simulink model "MultirotorSimPx4v1_8ContMatrix"  (R2018b)
settings: Solver=ode45  StartTime=0.0  StopTime=Simulation.T_END  MaxStep=Simulation.TS_MAX  RelTol=1e-3  EnableMultiTasking=on
PreLoadFcn:
  | % InitializeParameters;
undefined symbols (not defined in the file): Ctrl, Initial, Kpid, Uav, Wind
libraries: QuaternionLibrary x13, simulink x5, simulink_extras x4
(part 1 of 2)
settings Model: Creator=jban039  LastModifiedBy=jban039
settings DataIOCC: Decimation=10  ExternalInput=getinputstruct(op1(2))  InitialState=getstatestruct(op)  SaveFormat=StructureWithTime  ReturnWorkspaceOutputs=on  OutputTimes=Simulation.T_OUT
settings OptimizationCC: LifeSpan=inf
settings DebuggingCC: ReadBeforeWriteMsg=DisableAll  WriteAfterWriteMsg=DisableAll  WriteAfterReadMsg=DisableAll  MultiTaskDSMMsg=none  UnconnectedLineMsg=none  AllowSymbolicDim=off  SFUnexpectedBacktrackingDiag=warning  SFNoUnconditionalDefaultTransitionDiag=warning  SFExecutionAtInitializationDiag=none
settings ModelReferenceCC: UpdateModelReferenceTargets=IfOutOfDate  ModelReferenceMinAlgLoopOccurrences=on  PropagateSignalLabelsOutOfModel=off
settings SFSimCC: SFSimEcho=off  SimUseLocalCustomCode=off
settings RTWCC: RTWUseLocalCustomCode=off
settings CodeAppCC: StateflowObjectComments=on
settings GRTTargetCC: TargetLangStandard=C89/C90 (ANSI)
settings ConfigComp: CovMetricSettings=dw  CovHtmlReporting=on  CovSaveCumulativeToWorkspaceVar=on  CovSaveSingleToWorkspaceVar=on  CovExternalEMLEnable=off

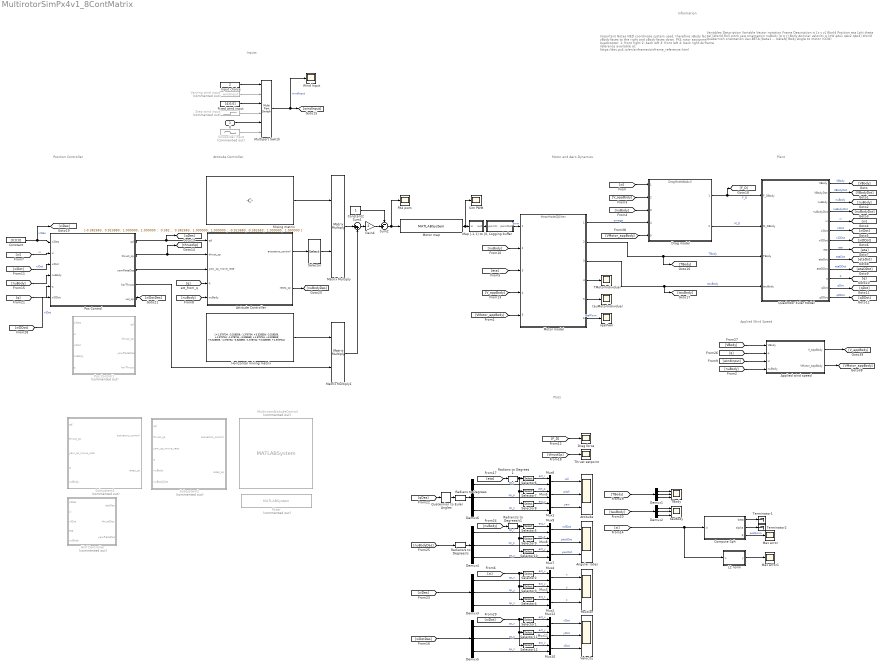
== system MultirotorSimPx4v1_8ContMatrix ==
  note: Plots
  note: Inputs
  note: Motor and Aero Dynamics
  note: Plant
  note: Attitude Controller
  note: Position Controller
  note: Applied Wind Speed
  note: Important Notes
      |
      | NED coordinate system used, therefore xBody faces forward, yBody faces to the right and zBody faces down.
      | PX4 rotor assignment for quadcopter:
      | 1: front right
      | 2: back left
      | 3: front left
      | 4: back right
      | Airframe reference available at:
      | https://dev.px4.io/en/airframes/airframe_reference.html
  note: Variables Description
      |
      | Variable
      | Vector notation
      | Frame
      | Description
      |
      | xi
      | [x y z]
      | World
      | Position
      |
      | eta
      | [phi theta psi]
      | World
      | Roll pitch yaw orientation
      |
      | nuBody
      | [p q r]
      | Body
      | Angular velocity
      |
      | q
      | [qW qAx1 qAx2 qAx3]
      | World
      | Quaternion orientation
      |
      | Uav.BETA
      | [beta1 ... betaN]
      | Body
      | Angle to motor (CCW)
  note: Information
  U : Inport  PortDimensions=3
  Angular rates : Scope  NumInputPorts=3
  Applied wind speed : Subsystem
  Attitude : Scope  NumInputPorts=3
  Attitude Controller : Subsystem
      mask Display: fprintf('MC_ATT_CONTROL\n\nCONTINUOUS')
  Compute Sph : MATLAB Function  TreatAsAtomicUnit=on
  Constant : Constant  Value=[0;0;0]
  Constant2 : Constant
  Demux{1..6} (6 alike) : Demux  Outputs=3
  Drag force : Scope
  Drag model : ModelReference  ModelNameDialog=DragModelAIAAv3  SimulationMode=Normal  ModelReferenceVersion=1.368
  Fixed wind input : Constant  Value=[4;0;0]
  Gain4 : Gain  Gain=2
  Hinf Controller : Subsystem  Commented=on
  Horizontal mixing matrix : Constant  Value=|
      | [+1.378734, -3.328559;
      |  -1.378734, +3.328559;
      |  -3.328559, +1.378734;
      |  -1.378734, -3.328559;
      |  +1.378734, +3.328559;
      |  +3.328559, -1.378734;
      |  -3.328559, -1.378734;
      |  +3.328559, +1.378734]
  Input choice : Constant  Value=2
  L2 norm : MATLAB Function  TreatAsAtomicUnit=on
  Logging buffer : Subsystem
  Map [-1,1] to [0,1] : Subsystem
  Matrix Multiply : Product  Multiplication=Matrix(*)
  Matrix Multiply1 : Product  Multiplication=Matrix(*)
  Max error : Scope
  Max error1 : Scope
  Mixer : MATLABSystem  Commented=on  SCDEnableBlockLinearizationSpecification=on  System=MultirotorMixer  airframeConfig=5  useHorThrust=0  outputSatStatus=0  SimulateUsing=Interpreted execution
      mask Type: MultirotorMixer
      mask Display:
      | disp(['MULTIROTOR' char(10) 'MIXER' char(10) 'octa_x']);
      | port_label('input',1,'actuatorsControl');
      | port_label('output',1,'px4PWM');
  Mixing matrix : Constant  Value=|
      | [-0.382683,  0.923880,  1.000000,  1.000000 ;
      |   0.382683, -0.923880,  1.000000,  1.000000 ;
      |  -0.923880,  0.382683, -1.000000,  1.000000 ;
      |  -0.382683, -0.923880, -1.000000,  1.000000 ;
      |   0.382683,  0.923880, -1.000000,  1.000000 ;
      |   0.923880, -0.382683, -1.000000,  1.000000 ;
      |   0.923880,  0.382683,  1.000000,  1.000000 ;
      |  -0.923880, -0.382683,  1.000000,  1.000000 ]
  Motor map : MATLABSystem  System=MotorMap  airframeConfig=5  SimulateUsing=Code generation
      mask Type: MotorMap
      mask Display:
      | disp(['MOTOR' char(10) 'MAP' char(10) 'octa_x']);
      | port_label('input',1,'px4PWM');
      | port_label('output',1,'simPWM');
  Motor model : ModelReference  ModelNameDialog=MotorModelZJChen  SimulationMode=Normal  ModelReferenceVersion=1.421
  Multiport Switch : MultiPortSwitch  Inputs=5
  MultirotorAttitudeControl : MATLABSystem  Commented=on  System=MulticopterAttitudeControl  acro_expo_rp=0.69  acro_expo_y=0.69  acro_pitch_max=720  acro_roll_max=720  acro_superexpo_rp=0.7  acro_superexpo_y=0.7  acro_yaw_max=540  airmode=0  d_term_cutoff_freq=30  pitch_rate_d=0.003  pitch_rate_ff=0  pitch_rate_i=0.05  pitch_rate_max=220  pitch_rate_p=0.15  pitch_p=6.5  pitch_rate_integ_lim=0.3  rattitude_thres=0.8  roll_rate_d=0.003  roll_rate_ff=0  roll_rate_i=0.05  roll_rate_max=220  roll_rate_p=0.15  roll_p=6.5  roll_rate_integ_lim=0.3  tpa_breakpoint_d=1  tpa_breakpoint_i=1  tpa_breakpoint_p=1  tpa_rate_d=0  tpa_rate_i=0  tpa_rate_p=0  yaw_rate_d=0  yaw_rate_ff=0  yaw_rate_i=0.1  yaw_rate_max=200  yaw_rate_p=0.2  yaw_auto_max=45  yaw_p=2.8  yaw_rate_integ_lim=0.3  man_throttle_min=0.08  man_tilt_max_deg=35  yaw_rate_scaling=200  throttle_hover=0.5  throttle_max=1  board_rotation_param=0  board_offset_x=0  board_offset_y=0  board_offset_z=0  bat_scale_en=0  throttle_curve=0  vehicle_status_is_rotary_wing=1  vehicle_status_is_vtol=0  loop_update_rate_hz=250  simple_mode=1  output_rates=0  SimulateUsing=Code generation
      mask Type: MulticopterAttitudeControl
      mask Display:
      | disp(['MulticopterAttitudeControl' char(10) '' char(10) 'v1.82']);
      | port_label('input',1,'qDes');
      | port_label('input',2,'thrustDes');
      | port_label('input',3,'yawRateDes');
      | port_label('input',4,'qMeasured');
      | port_label('input',5,'nuBody');
      | port_label('output',1,'actuatorsControl');
  Mux{1..12} (12 alike) : Mux  Inputs=2
  PX4 pwm : Scope
  Pos Control : Subsystem
      mask Display: fprintf('MC_POS_CONTROL\n\nCONTINUOUS')
  Pos Control1 : Subsystem  Commented=on
  Position : Scope  NumInputPorts=3
  Quadrotor Euler Model : Subsystem
  Quaternion to Euler Angles : QuaternionLibrary/Quaternion to Euler Angles
  "Radians to Degrees " : QuaternionLibrary/Radians to Degrees   SystemSampleTime=-1
  Radians to Degrees 1 : QuaternionLibrary/Radians to Degrees   SystemSampleTime=-1
  Radians/s to Degrees/s : QuaternionLibrary/Radians//s to Degrees//s  SystemSampleTime=-1
  Radians/s to Degrees/s1 : QuaternionLibrary/Radians//s to Degrees//s  SystemSampleTime=-1
  Selector : Selector  InputPortWidth=8  IndexOptions=Index vector (dialog)  Indices=[1:4]  OutputSizes=1
  Selector{1..2,5..6} (4 alike) : Selector  InputPortWidth=3  IndexOptions=Index vector (dialog)  Indices=1  OutputSizes=1
  Selector{4,8,10,12} (4 alike) : Selector  InputPortWidth=3  IndexOptions=Index vector (dialog)  Indices=3  OutputSizes=1
  Selector{3,7,9,11} (4 alike) : Selector  InputPortWidth=3  IndexOptions=Index vector (dialog)  Indices=2  OutputSizes=1
  Sim PWM : Scope
  Sinusoidal input : Sin  Commented=on  Amplitude=Wind.Ampl  Bias=Wind.Bias  Frequency=Wind.Freq  SampleTime=0
  Step wind input : Step  Commented=on  Time=Wind.StepTime  Before=Wind.StepInit  After=Wind.StepFinal  SampleTime=0
  Subsystem1 : Subsystem  Commented=on
  Subsystem2 : Subsystem  Commented=on
  Sum1 : Sum  Inputs=|++
  Sum2 : Sum  Inputs=-+|
  TBody : Scope  NumInputPorts=3
  TMotorIndividual : Scope
  Terminator1 : Terminator
  Terminator2 : Terminator
  Thrust setpoint : Scope
  Varying wind input : FromWorkspace  Commented=on  VariableName=windInput  SampleTime=0
  Velocity : Scope  NumInputPorts=3
  Wind Input : Scope
  realPwm : Scope
  tauBody : Scope  NumInputPorts=3
  tauMotorIndividual : Scope
  wires:
  Motor model/1 -> Drag model/4  "omega"
  Motor model/2 -> [TBody], Quadrotor Euler Model/3(TBody)  "TBody"
  Drag model/2 -> Quadrotor Euler Model/2(M_DBody)  "M_D"
  Quadrotor Euler Model/1(VBody) -> [VBody]  "VBody"
  Quadrotor Euler Model/2(VBodyDot) -> [VBodyDot]  "VBodyDot"
  Quadrotor Euler Model/3(nuBody) -> [nuBody]  "nuBody"
  Quadrotor Euler Model/4(nuBodyDot) -> [nuBodyDot]  "nuBodyDot"
  Quadrotor Euler Model/5(xi) -> [xi]  "xi"
  Quadrotor Euler Model/6(xiDot) -> [xiDot]  "xiDot"
  Quadrotor Euler Model/7(xiDDot) -> [xiDDot]  "xiDDot"
  Quadrotor Euler Model/8(eta) -> [eta]  "eta"
  Quadrotor Euler Model/9(etaDot) -> [etaDot]  "etaDot"
  Quadrotor Euler Model/10(etaDDot) -> [etaDDot]  "etaDDot"
  [V_appBody] -> Drag model/2
  [nuBody] -> Motor model/2
  Quadrotor Euler Model/11(q) -> [q]  "q"
  Quadrotor Euler Model/12(qDot) -> [qDot]  "qDot"
  Quadrotor Euler Model/13(qDDot) -> [qDDot]  "qDDot"
  Drag model/1 -> Quadrotor Euler Model/1(F_DBody), [F_D]  "F_D"
  Logging buffer/1(pwmOut) -> Motor model/1  "pwm"
  Sum2/1 -> PX4 pwm/1, Motor map/1
  [nuBody] -> Drag model/3
  [eta] -> Motor model/3
  [V_appBody] -> Motor model/4
  Motor model/4 -> TMotorIndividual/1
  Motor model/5 -> tauMotorIndividual/1
  [xi] -> Drag model/1
  [VMotor_appBody] -> Motor model/5
  [VMotor_appBody] -> Drag model/5
  Pos Control/1(qd) -> [qDes], Attitude Controller/1(qd)
  Motor model/3 -> [tauBody], Quadrotor Euler Model/4(tauBody)  "tauBody"
  [VBody] -> Applied wind speed/1(VBody)
  [q] -> Applied wind speed/2(q)
  [windInput] -> Applied wind speed/3(U)
  Applied wind speed/1(V_appBody) -> [V_appBody]
  Applied wind speed/2(VMotor_appBody) -> [VMotor_appBody]
  [nuBody] -> Applied wind speed/4(nuBody)
  Motor model/6 -> realPwm/1  "realPwm"
  [nuBody] -> Attitude Controller/5(nuBody)
  Motor map/1 -> Sim PWM/1, Map [-1,1] to [0,1]/1(in)
  Map [-1,1] to [0,1]/1(out) -> Logging buffer/1(pwmIn)
  Selector/1 -> Matrix Multiply/2
  Mixing matrix/1 -> Matrix Multiply/1
  Attitude Controller/1(actuators_control) -> Selector/1
  Gain4/1 -> Sum2/2
  Constant2/1 -> Sum2/1
  Matrix Multiply/1 -> Sum1/1
  Pos Control/2(thrust_sp) -> [thrustSp], Attitude Controller/2(thrust_sp)
  Pos Control/3(yawRateDes) -> Attitude Controller/3(yaw_sp_move_rate)
  [xiDot] -> Pos Control/3(xiDot)  "xiDot"
  [xi] -> Pos Control/2(xi)  "xi"
  [nuBody] -> Pos Control/4(nuBody)
  Constant/1 -> Pos Control/1(xiDes), [xiDes]  "xiDes"
  Attitude Controller/2(rates_sp) -> [nuBodyDes]
  [xi] -> L2 norm/1(u), Compute Sph/1(in)
  Mux1/1 -> Attitude/3  "yaw"
  [eta] -> Radians to Degrees 1/1
  Radians to Degrees 1/1 -> Selector6/1, Selector7/1, Selector8/1
  "Radians to Degrees "/1 -> Demux6/1
  Mux5/1 -> Attitude/2  "pitch"
  Mux6/1 -> Attitude/1  "roll"
  [qDes] -> Quaternion to Euler Angles/1
  Selector8/1 -> Mux1/1  "act_y"
  Demux6/2 -> Mux5/2  "sp_p"
  Demux6/1 -> Mux6/2  "sp_r"
  Quaternion to Euler Angles/1 -> "Radians to Degrees "/1
  Selector7/1 -> Mux5/1  "act_p"
  Selector6/1 -> Mux6/1  "act_r"
  Demux6/3 -> Mux1/2  "sp_y"
  Matrix Multiply1/1 -> Sum1/2
  Horizontal mixing matrix/1 -> Matrix Multiply1/1
  Pos Control/4(horThrust) -> Matrix Multiply1/2
  [thrustSp] -> Thrust setpoint/1
  Varying wind input/1 -> Multiport Switch/2
  Fixed wind input/1 -> Multiport Switch/3
  Multiport Switch/1 -> Wind Input/1, [windInput]  "windInput"
  Demux1/3 -> TBody/3
  Demux1/2 -> TBody/2
  [TBody] -> Demux1/1
  Demux1/1 -> TBody/1
  Demux2/1 -> tauBody/1
  [tauBody] -> Demux2/1
  Demux2/2 -> tauBody/2
  Demux2/3 -> tauBody/3
  Step wind input/1 -> Multiport Switch/4
  Input choice/1 -> Multiport Switch/1
  [q] -> Attitude Controller/4(q)
  [q] -> Pos Control/5(q)
  Sum1/1 -> Gain4/1
  Compute Sph/1(beta) -> Terminator1/1
  Compute Sph/2(alpha) -> Terminator2/1
  Compute Sph/3(R) -> Max error/1  "posNorm"
  U/1 -> Multiport Switch/5
  [F_D] -> Drag force/1
  Sinusoidal input/1 -> Multiport Switch/6
  L2 norm/1(y) -> Max error1/1
  Demux3/3 -> Mux2/2  "sp_z"
  Selector2/1 -> Mux4/1  "act_x"
  Selector3/1 -> Mux3/1  "act_y"
  Demux3/1 -> Mux4/2  "sp_x"
  Demux3/2 -> Mux3/2  "sp_y"
  Selector4/1 -> Mux2/1  "act_z"
  Mux4/1 -> Position/1  "x"
  Mux3/1 -> Position/2  "y"
  [xiDes] -> Demux3/1
  [xi] -> Selector4/1, Selector3/1, Selector2/1
  Mux2/1 -> Position/3  "z"
  Demux4/3 -> Mux7/2  "sp_y"
  Selector5/1 -> Mux9/1  "act_r"
  Selector9/1 -> Mux8/1  "act_p"
  [nuBodyDes] -> Radians/s to Degrees/s/1
  Demux4/1 -> Mux9/2  "sp_r"
  Demux4/2 -> Mux8/2  "sp_p"
  Selector10/1 -> Mux7/1  "act_y"
  Mux9/1 -> Angular rates/1  "rollDot"
  Mux8/1 -> Angular rates/2  "pitchDot"
  Radians/s to Degrees/s/1 -> Demux4/1
  Radians/s to Degrees/s1/1 -> Selector10/1, Selector9/1, Selector5/1
  [nuBody] -> Radians/s to Degrees/s1/1
  Mux7/1 -> Angular rates/3  "yawDot"
  Pos Control/5(vel_sp) -> [xiDotDes]
  Mux10/1 -> Velocity/3  "zDot"
  [xiDot] -> Selector1/1, Selector11/1, Selector12/1
  [xiDotDes] -> Demux5/1
  Mux11/1 -> Velocity/2  "yDot"
  Mux12/1 -> Velocity/1  "xDot"
  Selector12/1 -> Mux10/1  "act_z"
  Demux5/2 -> Mux11/2  "sp_y"
  Demux5/1 -> Mux12/2  "sp_x"
  Selector11/1 -> Mux11/1  "act_y"
  Selector1/1 -> Mux12/1  "act_x"
  Demux5/3 -> Mux10/2  "sp_z"
  [xiDDot] -> Pos Control/6(xiDDot)  "xiDot"

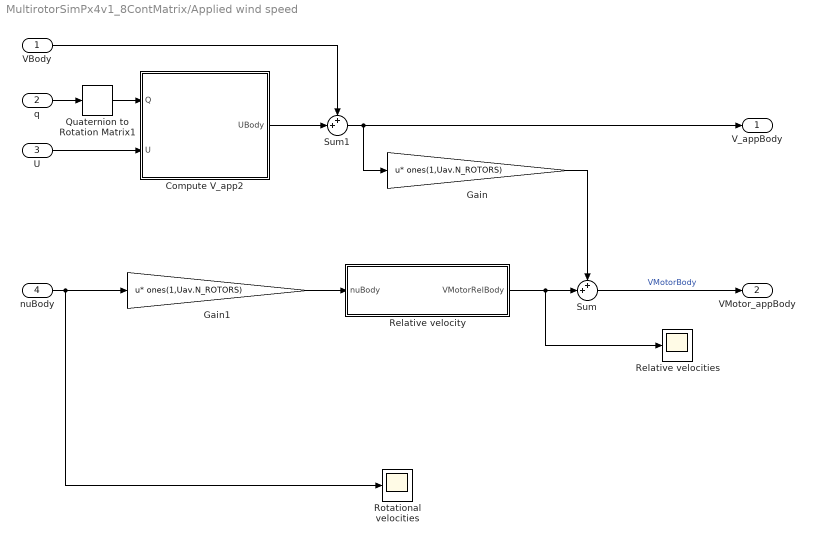
== system MultirotorSimPx4v1_8ContMatrix/Applied wind speed ==
  VBody : Inport  Unit=m/s
  q : Inport  Port=2
  U : Inport  Port=3  Unit=m/s
  nuBody : Inport  Port=4  Unit=rad/s
  Compute V_app2 : MATLAB Function  TreatAsAtomicUnit=on
  Gain : Gain  Gain=ones(1,Uav.N_ROTORS)  Multiplication=Matrix(u*K)
  Gain1 : Gain  Gain=ones(1,Uav.N_ROTORS)  Multiplication=Matrix(u*K)
  Quaternion to Rotation Matrix1 : QuaternionLibrary/Quaternion to Rotation Matrix
  Relative velocities : Scope
  Relative velocity : MATLAB Function  TreatAsAtomicUnit=on
  Rotational velocities : Scope
  Sum : Sum  Inputs=++|
  Sum1 : Sum  Inputs=++|
  V_appBody : Outport  Unit=m/s
  VMotor_appBody : Outport  Port=2  Unit=m/s  PortDimensions=[3,Uav.N_ROTORS]
  wires:
  U/1 -> Compute V_app2/2(U)
  Sum/1 -> VMotor_appBody/1  "VMotorBody"
  Quaternion to Rotation Matrix1/1 -> Compute V_app2/1(Q)
  nuBody/1 -> Gain1/1, Rotational velocities/1
  Gain/1 -> Sum/1
  VBody/1 -> Sum1/1
  q/1 -> Quaternion to Rotation Matrix1/1
  Relative velocity/1(VMotorRelBody) -> Relative velocities/1, Sum/2
  Compute V_app2/1(UBody) -> Sum1/2
  Sum1/1 -> Gain/1, V_appBody/1
  Gain1/1 -> Relative velocity/1(nuBody)

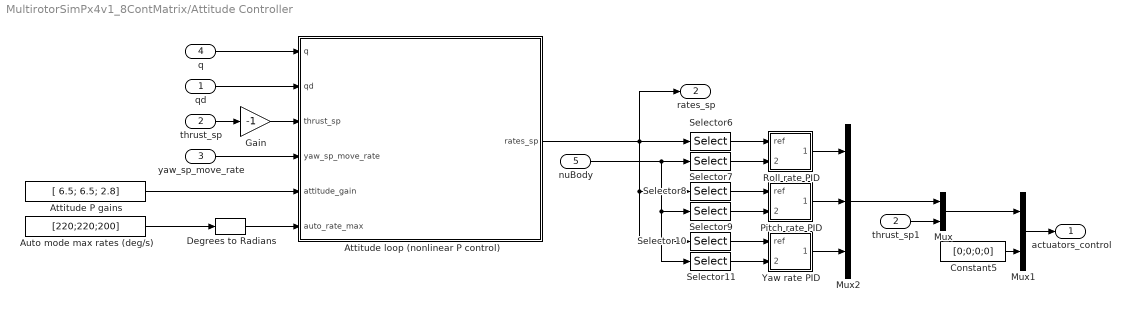
== system MultirotorSimPx4v1_8ContMatrix/Attitude Controller ==
  qd : Inport
  thrust_sp : Inport  Port=2  PortDimensions=1
  yaw_sp_move_rate : Inport  Port=3  Unit=rad/s
  q : Inport  Port=4
  nuBody : Inport  Port=5  Unit=rad/s
  Attitude P gains : Constant  Value=[ 6.5; 6.5; 2.8]
  Attitude loop (nonlinear P control) : MATLAB Function  TreatAsAtomicUnit=on
  Auto mode max rates (deg/s) : Constant  Value=[220;220;200]
  Constant5 : Constant  Value=[0;0;0;0]
  Degrees to Radians : simulink_extras/Transformations/Degrees to Radians
  Gain : Gain  Gain=-1
  Mux : Mux  Inputs=2
  Mux1 : Mux  Inputs=2
  Mux2 : Mux  Inputs=3
  Pitch rate PID : Subsystem  mask{PID_P=0.15, PID_I=0.05, PID_D=0.003, PID_FC=30, PID_I_STATENAME='AttRatePID_I_pitch', PID_D_STATENAME='AttRatePID_D_pitch'}
      mask prompts: PID_P "P gain"; PID_I "I gain"; PID_D "D gain"; PID_FC "D filter cutoff (Hz)"; PID_I_STATENAME "Integartor state name"; PID_D_STATENAME "D filter state name"
      mask DialogControl DescGroupVar Prompt: PID Controller with Second Order Derivative Filter
      mask DialogControl DescTextVar Prompt: The derivative gain is applied on the derivative of y rather than that of the error (r-y).
      mask Display:
      | disp('PID(s)')
      | port_label('input', 1, 'r')
      | port_label('input', 2, 'y')
      | text(1,0,'2^{nd}','horizontalAlignment','right','interpreter','tex','verticalAlignment','bottom')
  Roll rate PID : Subsystem  mask{PID_P=0.15, PID_I=0.05, PID_D=0.003, PID_FC=30, PID_I_STATENAME='AttRatePID_I_roll', PID_D_STATENAME='AttRatePID_D_roll'}
      mask prompts: PID_P "P gain"; PID_I "I gain"; PID_D "D gain"; PID_FC "D filter cutoff (Hz)"; PID_I_STATENAME "Integartor state name"; PID_D_STATENAME "D filter state name"
      mask DialogControl DescGroupVar Prompt: PID Controller with Second Order Derivative Filter
      mask DialogControl DescTextVar Prompt: The derivative gain is applied on the derivative of y rather than that of the error (r-y).
      mask Display:
      | disp('PID(s)')
      | port_label('input', 1, 'r')
      | port_label('input', 2, 'y')
      | text(1,0,'2^{nd}','horizontalAlignment','right','interpreter','tex','verticalAlignment','bottom')
  Selector10 : Selector  InputPortWidth=3  IndexOptions=Index vector (dialog)  Indices=3  OutputSizes=1
  Selector11 : Selector  InputPortWidth=3  IndexOptions=Index vector (dialog)  Indices=3  OutputSizes=1
  Selector6 : Selector  InputPortWidth=3  IndexOptions=Index vector (dialog)  Indices=1  OutputSizes=1
  Selector7 : Selector  InputPortWidth=3  IndexOptions=Index vector (dialog)  Indices=1  OutputSizes=1
  Selector8 : Selector  InputPortWidth=3  IndexOptions=Index vector (dialog)  Indices=2  OutputSizes=1
  Selector9 : Selector  InputPortWidth=3  IndexOptions=Index vector (dialog)  Indices=2  OutputSizes=1
  Yaw rate PID : Subsystem  mask{PID_P=0.2, PID_I=0.1, PID_D=0, PID_FC=30, PID_I_STATENAME='AttRatePID_I_yaw', PID_D_STATENAME='AttRatePID_D_yaw'}
      mask prompts: PID_P "P gain"; PID_I "I gain"; PID_D "D gain"; PID_FC "D filter cutoff (Hz)"; PID_I_STATENAME "Integartor state name"; PID_D_STATENAME "D filter state name"
      mask DialogControl DescGroupVar Prompt: PID Controller with Second Order Derivative Filter
      mask DialogControl DescTextVar Prompt: The derivative gain is applied on the derivative of y rather than that of the error (r-y).
      mask Display:
      | disp('PID(s)')
      | port_label('input', 1, 'r')
      | port_label('input', 2, 'y')
      | text(1,0,'2^{nd}','horizontalAlignment','right','interpreter','tex','verticalAlignment','bottom')
  thrust_sp1 : InportShadow  Port=2  PortDimensions=1
  actuators_control : Outport  PortDimensions=8
  rates_sp : Outport  Port=2  Unit=rad/s
  wires:
  nuBody/1 -> Selector7/1, Selector9/1, Selector11/1
  Selector9/1 -> Pitch rate PID/2(meas)
  Selector11/1 -> Yaw rate PID/2(meas)
  Selector10/1 -> Yaw rate PID/1(ref)
  Selector8/1 -> Pitch rate PID/1(ref)
  Selector7/1 -> Roll rate PID/2(meas)
  Selector6/1 -> Roll rate PID/1(ref)
  Mux2/1 -> Mux/1
  Pitch rate PID/1(Out) -> Mux2/2
  Roll rate PID/1(Out) -> Mux2/1
  Yaw rate PID/1(Out) -> Mux2/3
  qd/1 -> Attitude loop (nonlinear P control)/2(qd)
  q/1 -> Attitude loop (nonlinear P control)/1(q)
  Attitude P gains/1 -> Attitude loop (nonlinear P control)/5(attitude_gain)
  Auto mode max rates (deg/s)/1 -> Degrees to Radians/1
  Degrees to Radians/1 -> Attitude loop (nonlinear P control)/6(auto_rate_max)
  yaw_sp_move_rate/1 -> Attitude loop (nonlinear P control)/4(yaw_sp_move_rate)
  Mux/1 -> Mux1/1
  Constant5/1 -> Mux1/2
  Mux1/1 -> actuators_control/1
  thrust_sp/1 -> Gain/1
  Attitude loop (nonlinear P control)/1(rates_sp) -> Selector6/1, Selector8/1, Selector10/1, rates_sp/1
  Gain/1 -> Attitude loop (nonlinear P control)/3(thrust_sp)
  thrust_sp1/1 -> Mux/2

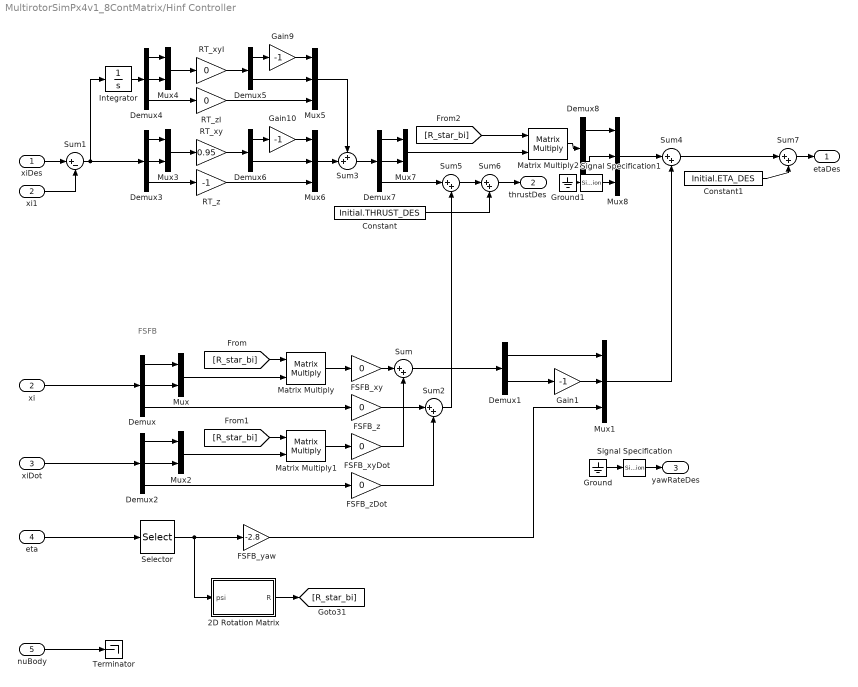
== system MultirotorSimPx4v1_8ContMatrix/Hinf Controller ==
  note: FSFB
  xiDes : Inport  PortDimensions=3
  xi : Inport  Port=2
  xiDot : Inport  Port=3
  eta : Inport  Port=4
  nuBody : Inport  Port=5
  2D Rotation Matrix : Subsystem
  Constant : Constant  Value=Initial.THRUST_DES
  Constant1 : Constant  Value=Initial.ETA_DES
  Demux{,2..4,7} (5 alike) : Demux  Outputs=3
  Demux{1,5..6,8} (4 alike) : Demux  Outputs=2
  FSFB_xy : Gain  Gain=0
  FSFB_xyDot : Gain  Gain=0
  FSFB_yaw : Gain  Gain=-2.8
  FSFB_z : Gain  Gain=0
  FSFB_zDot : Gain  Gain=0
  Gain1 : Gain  Gain=-1
  Gain10 : Gain  Gain=-1
  Gain9 : Gain  Gain=-1
  Ground : Ground
  Ground1 : Ground
  Integrator : Integrator  ContinuousStateAttributes='POS_CTRL_I'
  Matrix Multiply : Product  Multiplication=Matrix(*)
  Matrix Multiply1 : Product  Multiplication=Matrix(*)
  Matrix Multiply2 : Product  Multiplication=Matrix(*)
  Mux{,2..4,7} (5 alike) : Mux  Inputs=2
  Mux{1,5..6,8} (4 alike) : Mux  Inputs=3
  RT_xy : Gain  Gain=0.95
  RT_xyI : Gain  Gain=0
  RT_z : Gain  Gain=-1
  RT_zI : Gain  Gain=0
  Selector : Selector  InputPortWidth=3  IndexOptions=Index vector (dialog)  Indices=3  OutputSizes=1
  Signal Specification : SignalSpecification  Dimensions=1
  Signal Specification1 : SignalSpecification  Dimensions=1
  Sum{,2,4..7} (6 alike) : Sum  Inputs=|++
  Sum1 : Sum  Inputs=|+-
  Sum3 : Sum  Inputs=++|
  Terminator : Terminator
  xi1 : InportShadow  Port=2
  etaDes : Outport
  thrustDes : Outport  Port=2
  yawRateDes : Outport  Port=3
  wires:
  FSFB_xy/1 -> Sum/1
  Mux/1 -> Matrix Multiply/2
  Demux/1 -> Mux/1
  Demux/2 -> Mux/2
  Demux2/2 -> Mux2/2
  Demux2/1 -> Mux2/1
  Matrix Multiply1/1 -> FSFB_xyDot/1
  FSFB_xyDot/1 -> Sum/2
  Demux2/3 -> FSFB_zDot/1
  Demux/3 -> FSFB_z/1
  Sum/1 -> Demux1/1
  2D Rotation Matrix/1(R) -> [R_star_bi]
  Matrix Multiply/1 -> FSFB_xy/1
  eta/1 -> Selector/1
  Selector/1 -> FSFB_yaw/1, 2D Rotation Matrix/1(psi)
  [R_star_bi] -> Matrix Multiply/1
  [R_star_bi] -> Matrix Multiply1/1
  Mux2/1 -> Matrix Multiply1/2
  FSFB_z/1 -> Sum2/1
  FSFB_zDot/1 -> Sum2/2
  Demux1/1 -> Mux1/1
  Demux1/2 -> Gain1/1
  Sum2/1 -> Sum5/2
  FSFB_yaw/1 -> Mux1/3
  Mux1/1 -> Sum4/2
  Ground/1 -> Signal Specification/1
  nuBody/1 -> Terminator/1
  xiDes/1 -> Sum1/1
  xi1/1 -> Sum1/2
  Sum1/1 -> Integrator/1, Demux3/1
  Demux3/1 -> Mux3/1
  Demux3/2 -> Mux3/2
  Mux3/1 -> RT_xy/1
  Demux3/3 -> RT_z/1
  Demux4/3 -> RT_zI/1
  Mux4/1 -> RT_xyI/1
  Demux4/2 -> Mux4/2
  Demux4/1 -> Mux4/1
  Integrator/1 -> Demux4/1
  RT_xyI/1 -> Demux5/1
  Demux5/1 -> Gain9/1
  RT_zI/1 -> Mux5/3
  RT_z/1 -> Mux6/3
  Demux6/1 -> Gain10/1
  RT_xy/1 -> Demux6/1
  Mux6/1 -> Sum3/2
  Mux5/1 -> Sum3/1
  Sum3/1 -> Demux7/1
  Demux7/1 -> Mux7/1
  Demux7/2 -> Mux7/2
  Demux7/3 -> Sum5/1
  [R_star_bi] -> Matrix Multiply2/1
  Mux7/1 -> Matrix Multiply2/2
  Matrix Multiply2/1 -> Demux8/1
  Demux8/2 -> Mux8/2
  Demux8/1 -> Mux8/1
  Ground1/1 -> Signal Specification1/1
  Mux8/1 -> Sum4/1
  Sum5/1 -> Sum6/1
  Sum4/1 -> Sum7/1
  Demux5/2 -> Mux5/2
  Demux6/2 -> Mux6/2
  Gain1/1 -> Mux1/2
  Signal Specification/1 -> yawRateDes/1
  Signal Specification1/1 -> Mux8/3
  xi/1 -> Demux/1
  xiDot/1 -> Demux2/1
  Gain10/1 -> Mux6/1
  Gain9/1 -> Mux5/1
  Sum6/1 -> thrustDes/1
  Constant/1 -> Sum6/2
  Sum7/1 -> etaDes/1
  Constant1/1 -> Sum7/2

== system MultirotorSimPx4v1_8ContMatrix/Logging buffer ==
  pwmIn : Inport
  Rate Transition : RateTransition  Commented=through  SCDEnableBlockLinearizationSpecification=on
  pwmOut : Outport
  wires:
  pwmIn/1 -> Rate Transition/1
  Rate Transition/1 -> pwmOut/1

== system MultirotorSimPx4v1_8ContMatrix/Map [-1,1] to [0,1] ==
  in : Inport
  Constant : Constant
  Gain4 : Gain  Gain=0.5
  Sum : Sum  Inputs=++|
  out : Outport
  wires:
  Sum/1 -> Gain4/1
  Gain4/1 -> out/1
  in/1 -> Sum/2
  Constant/1 -> Sum/1

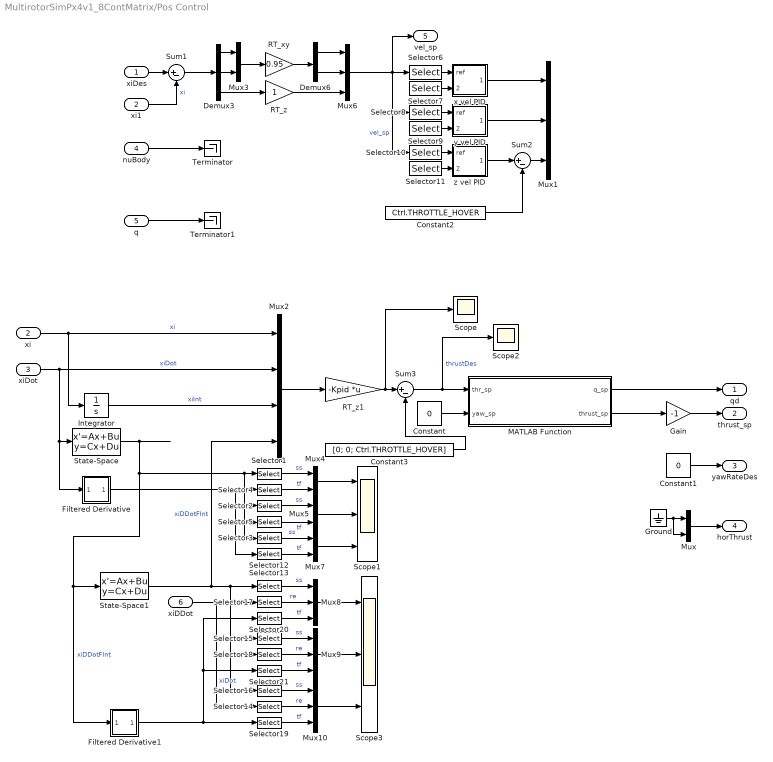
== system MultirotorSimPx4v1_8ContMatrix/Pos Control ==
  xiDes : Inport  Unit=m  PortDimensions=3
  xi : Inport  Port=2  Unit=m  PortDimensions=3
  xiDot : Inport  Port=3  Unit=m/s  PortDimensions=3
  nuBody : Inport  Port=4  Unit=rad/s
  q : Inport  Port=5
  xiDDot : Inport  Port=6  Unit=m/s^2  PortDimensions=3
  Constant : Constant  Value=0
  Constant1 : Constant  Value=0
  Constant2 : Constant  Value=Ctrl.THROTTLE_HOVER
  Constant3 : Constant  Value=[0; 0; Ctrl.THROTTLE_HOVER]
  Demux3 : Demux  Outputs=3
  Demux6 : Demux  Outputs=2
  Filtered Derivative : Subsystem  mask{PID_FC=5}
      mask prompts: PID_FC "D filter cutoff"
      mask Display: disp('s')
  Filtered Derivative1 : Subsystem  mask{PID_FC=5}
      mask prompts: PID_FC "D filter cutoff"
      mask Display: disp('s')
  Gain : Gain  Gain=-1
  Ground : Ground
  Integrator : Integrator  ContinuousStateAttributes='xiInt'
  MATLAB Function : MATLAB Function  TreatAsAtomicUnit=on
  Mux{,3..5,7} (5 alike) : Mux  Inputs=2
  Mux{1,6,8..10} (5 alike) : Mux  Inputs=3
  Mux2 : Mux
  RT_xy : Gain  Gain=0.95
  RT_z : Gain
  RT_z1 : Gain  Gain=-Kpid  Multiplication=Matrix(K*u)
  Scope : Scope
  Scope1 : Scope  NumInputPorts=3
  Scope2 : Scope
  Scope3 : Scope  NumInputPorts=3
  Selector{1,4,6..7,13,17,20} (7 alike) : Selector  InputPortWidth=3  IndexOptions=Index vector (dialog)  Indices=1  OutputSizes=1
  Selector{3,10..12,14,16,19} (7 alike) : Selector  InputPortWidth=3  IndexOptions=Index vector (dialog)  Indices=3  OutputSizes=1
  Selector{2,5,8..9,15,18,21} (7 alike) : Selector  InputPortWidth=3  IndexOptions=Index vector (dialog)  Indices=2  OutputSizes=1
  State-Space : StateSpace  A=-(PID_FC*2*pi) .* eye(3)  B=(PID_FC*2*pi) .* eye(3)  C=eye(3)  D=zeros(3)  InitialCondition=0  ContinuousStateAttributes='xiDDotFInt'  mask{PID_FC=5}
      mask prompts: PID_FC "Filter cutoff frequency"
  State-Space1 : StateSpace  A=-(PID_FC*2*pi) .* eye(3)  B=(PID_FC*2*pi) .* eye(3)  C=-(PID_FC*2*pi) .* eye(3)  D=(PID_FC*2*pi) .* eye(3)  InitialCondition=0  ContinuousStateAttributes='xiDDotFInt'  mask{PID_FC=5}
      mask prompts: PID_FC "Filter cutoff frequency"
  Sum1 : Sum  Inputs=|+-
  Sum2 : Sum  Inputs=|+-
  Sum3 : Sum  Inputs=|+-
  Terminator : Terminator
  Terminator1 : Terminator
  x vel PID : Subsystem  mask{PID_P=0.09, PID_I=0.02, PID_D=0.01, PID_FC=5, PID_I_STATENAME='velPID_I_x', PID_D_STATENAME='velPID_D_x'}
      mask prompts: PID_P "P gain"; PID_I "I gain"; PID_D "D gain"; PID_FC "D filter cutoff (Hz)"; PID_I_STATENAME "Integartor state name"; PID_D_STATENAME "D filter state name"
      mask DialogControl DescGroupVar Prompt: PID Controller with First Order Derivative Filter
      mask DialogControl DescTextVar Prompt: The derivative gain is applied on the derivative of y rather than that of the error (r-y).
      mask Display:
      | disp('PID(s)')
      | port_label('input', 1, 'r')
      | port_label('input', 2, 'y')
      | text(1,0,'1^{st}','horizontalAlignment','right','interpreter','tex','verticalAlignment','bottom')
  xi1 : InportShadow  Port=2  Unit=m  PortDimensions=3
  y vel PID : Subsystem  mask{PID_P=0.09, PID_I=0.02, PID_D=0.01, PID_FC=5, PID_I_STATENAME='velPID_I_y', PID_D_STATENAME='velPID_D_y'}
      mask prompts: PID_P "P gain"; PID_I "I gain"; PID_D "D gain"; PID_FC "D filter cutoff (Hz)"; PID_I_STATENAME "Integartor state name"; PID_D_STATENAME "D filter state name"
      mask DialogControl DescGroupVar Prompt: PID Controller with First Order Derivative Filter
      mask DialogControl DescTextVar Prompt: The derivative gain is applied on the derivative of y rather than that of the error (r-y).
      mask Display:
      | disp('PID(s)')
      | port_label('input', 1, 'r')
      | port_label('input', 2, 'y')
      | text(1,0,'1^{st}','horizontalAlignment','right','interpreter','tex','verticalAlignment','bottom')
  z vel PID : Subsystem  mask{PID_P=0.2, PID_I=0.1, PID_D=0, PID_FC=5, PID_I_STATENAME='velPID_I_z', PID_D_STATENAME='velPID_D_z'}
      mask prompts: PID_P "P gain"; PID_I "I gain"; PID_D "D gain"; PID_FC "D filter cutoff (Hz)"; PID_I_STATENAME "Integartor state name"; PID_D_STATENAME "D filter state name"
      mask DialogControl DescGroupVar Prompt: PID Controller with First Order Derivative Filter
      mask DialogControl DescTextVar Prompt: The derivative gain is applied on the derivative of y rather than that of the error (r-y).
      mask Display:
      | disp('PID(s)')
      | port_label('input', 1, 'r')
      | port_label('input', 2, 'y')
      | text(1,0,'1^{st}','horizontalAlignment','right','interpreter','tex','verticalAlignment','bottom')
  qd : Outport
  thrust_sp : Outport  Port=2
  yawRateDes : Outport  Port=3  Unit=rad/s
  horThrust : Outport  Port=4  PortDimensions=2
  vel_sp : Outport  Port=5  Unit=m/s
  wires:
  MATLAB Function/1(q_sp) -> qd/1
  Demux6/1 -> Mux6/1
  Constant1/1 -> yawRateDes/1
  Demux6/2 -> Mux6/2
  RT_xy/1 -> Demux6/1
  Demux3/3 -> RT_z/1
  Mux3/1 -> RT_xy/1
  Demux3/2 -> Mux3/2
  Demux3/1 -> Mux3/1
  xi1/1 -> Sum1/2  "xi"
  xiDes/1 -> Sum1/1
  nuBody/1 -> Terminator/1
  Sum3/1 -> Scope2/1, MATLAB Function/1(thr_sp)  "thrustDes"
  Constant/1 -> MATLAB Function/2(yaw_sp)
  RT_z/1 -> Mux6/3
  Constant2/1 -> Sum2/2
  Sum2/1 -> Mux1/3
  Gain/1 -> thrust_sp/1
  Sum1/1 -> Demux3/1
  x vel PID/1(Out) -> Mux1/1
  y vel PID/1(Out) -> Mux1/2
  z vel PID/1(Out) -> Sum2/1
  MATLAB Function/2(thrust_sp) -> Gain/1
  Ground/1 -> Mux/2, Mux/1
  Mux/1 -> horThrust/1
  q/1 -> Terminator1/1
  Selector11/1 -> z vel PID/2(meas)
  Selector10/1 -> z vel PID/1(ref)
  Selector9/1 -> y vel PID/2(meas)
  Selector8/1 -> y vel PID/1(ref)
  Selector7/1 -> x vel PID/2(meas)
  Selector6/1 -> x vel PID/1(ref)
  ? -> Selector11/1, Selector9/1, Selector7/1
  Mux6/1 -> vel_sp/1, Selector6/1, Selector8/1, Selector10/1  "vel_sp"
  xi/1 -> Integrator/1, Mux2/1  "xi"
  xiDot/1 -> Filtered Derivative/1(xiDot), State-Space/1, Mux2/2  "xiDot"
  State-Space/1 -> Filtered Derivative1/1(xiDot), State-Space1/1, Selector3/1, Selector2/1, Selector1/1  "xiDDotFInt"
  Integrator/1 -> Mux2/3  "xiInt"
  Mux2/1 -> RT_z1/1
  RT_z1/1 -> Scope/1, Sum3/1
  Constant3/1 -> Sum3/2
  Mux4/1 -> Scope1/1
  Filtered Derivative/1(xiDDotF) -> Selector12/1, Selector5/1, Selector4/1
  Selector1/1 -> Mux4/1  "ss"
  Selector4/1 -> Mux4/2  "tf"
  Selector5/1 -> Mux5/2  "tf"
  Selector2/1 -> Mux5/1  "ss"
  Selector12/1 -> Mux7/2  "tf"
  Selector3/1 -> Mux7/1  "ss"
  Mux5/1 -> Scope1/2
  Mux7/1 -> Scope1/3
  Mux10/1 -> Scope3/3
  Mux9/1 -> Scope3/2
  Selector16/1 -> Mux10/1  "ss"
  Selector14/1 -> Mux10/2  "re"
  Selector15/1 -> Mux9/1  "ss"
  Selector18/1 -> Mux9/2  "re"
  Selector17/1 -> Mux8/2  "re"
  Selector13/1 -> Mux8/1  "ss"
  Mux8/1 -> Scope3/1
  xiDDot/1 -> Selector14/1, Selector18/1, Selector17/1  "xiDot"
  State-Space1/1 -> Mux2/4, Selector15/1, Selector16/1, Selector13/1  "xiDDotFInt"
  Filtered Derivative1/1(xiDDotF) -> Selector19/1, Selector21/1, Selector20/1
  Selector21/1 -> Mux9/3  "tf"
  Selector20/1 -> Mux8/3  "tf"
  Selector19/1 -> Mux10/3  "tf"

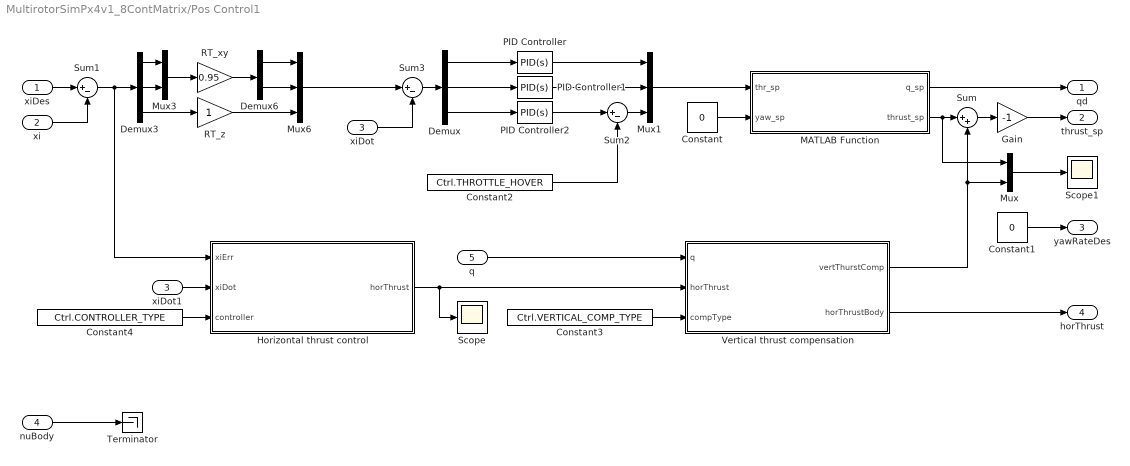
== system MultirotorSimPx4v1_8ContMatrix/Pos Control1 ==
  xiDes : Inport  PortDimensions=3
  xi : Inport  Port=2  PortDimensions=3
  xiDot : Inport  Port=3  PortDimensions=3
  nuBody : Inport  Port=4
  q : Inport  Port=5
  Constant : Constant  Value=0
  Constant1 : Constant  Value=0
  Constant2 : Constant  Value=Ctrl.THROTTLE_HOVER
  Constant3 : Constant  Value=Ctrl.VERTICAL_COMP_TYPE
  Constant4 : Constant  Value=Ctrl.CONTROLLER_TYPE
  Demux : Demux  Outputs=3
  Demux3 : Demux  Outputs=3
  Demux6 : Demux  Outputs=2
  Gain : Gain  Gain=-1
  Horizontal thrust control : Subsystem
  MATLAB Function : MATLAB Function  TreatAsAtomicUnit=on
  Mux : Mux  Inputs=2
  Mux1 : Mux  Inputs=3
  Mux3 : Mux  Inputs=2
  Mux6 : Mux  Inputs=3
  PID Controller : simulink/Continuous/PID Controller  Controller=PID  Form=Parallel  TimeDomain=Continuous-time  SampleTime=0.02  IntegratorMethod=Forward Euler  FilterMethod=Forward Euler  ControllerParametersSource=internal  P=0.09  I=0.02  D=0.01  UseFilter=on  N=100  TunerSelectOption=Transfer Function Based (PID Tuner App)  InitialConditionSource=internal  InitialConditionForIntegrator=0  InitialConditionForFilter=0  DifferentiatorICPrevScaledInput=0  ExternalReset=none  TrackingMode=off  Kt=1  LimitOutput=off  UpperSaturationLimit=inf  LowerSaturationLimit=-inf  LinearizeAsGain=on  AntiWindupMode=none  Kb=1  POutMin=[]  POutMax=[]  IOutMin=[]  IOutMax=[]  DOutMin=[]  DOutMax=[]  NOutMin=[]  NOutMax=[]  SumOutMin=[]  SumOutMax=[]  SaturationOutMin=[]  SaturationOutMax=[]  PParamMin=[]  PParamMax=[]  IParamMin=[]  IParamMax=[]  DParamMin=[]  DParamMax=[]  NParamMin=[]  NParamMax=[]  KbParamMin=[]  KbParamMax=[]  KtParamMin=[]  KtParamMax=[]  KbOutMin=[]  KbOutMax=[]  KtOutMin=[]  KtOutMax=[]  IntegratorOutMin=[]  IntegratorOutMax=[]  FilterOutMin=[]  FilterOutMax=[]  SumI1OutMin=[]  SumI1OutMax=[]  SumI2OutMin=[]  SumI2OutMax=[]  SumI3OutMin=[]  SumI3OutMax=[]  SumI4OutMin=[]  SumI4OutMax=[]  SumDOutMin=[]  SumDOutMax=[]  DifferentiatorOutMin=[]  DifferentiatorOutMax=[]  FilterDiffOutCoefMin=[]  FilterDiffOutCoefMax=[]  ReciprocalOutMin=[]  ReciprocalOutMax=[]  SumDenOutMin=[]  SumDenOutMax=[]  SumNumOutMin=[]  SumNumOutMax=[]  DivideOutMin=[]  DivideOutMax=[]  IntegratorContinuousStateAttributes=''  IntegratorStateMustResolveToSignalObject=off  IntegratorRTWStateStorageClass=Auto  FilterContinuousStateAttributes=''  FilterStateMustResolveToSignalObject=off  FilterRTWStateStorageClass=Auto  ParallelPVariant=InternalParameters  IdealPVariant=Disabled  IVariant=InternalParameters  DVariant=InternalParameters  IntegratorVariant=Continuous  SatVariant=Disabled  AWVariant=Passthrough  PCopyVariant=Disabled  TRVariant=Disabled  FdbkBlocksVariant=Forward  IdealPFdbkVariant=Disabled  SatFdbkVariant=Disabled  DerivativeFilterVariant=ContFilter  NVariant=InternalParameters  NCopyVariant=Disabled  FilterICVariant=InternalICsFilter  IntegratorICVariant=InternalICs  ExternalResetVariant=Disabled  TRSumVariant=Passthrough  SumFdbkVariant=Disabled  SumVariant=Sum_PID
  PID Controller1 : simulink/Continuous/PID Controller  Controller=PID  Form=Parallel  TimeDomain=Continuous-time  SampleTime=0.02  IntegratorMethod=Forward Euler  FilterMethod=Forward Euler  ControllerParametersSource=internal  P=0.09  I=0.02  D=0.01  UseFilter=on  N=100  TunerSelectOption=Transfer Function Based (PID Tuner App)  InitialConditionSource=internal  InitialConditionForIntegrator=0  InitialConditionForFilter=0  DifferentiatorICPrevScaledInput=0  ExternalReset=none  TrackingMode=off  Kt=1  LimitOutput=off  UpperSaturationLimit=inf  LowerSaturationLimit=-inf  LinearizeAsGain=on  AntiWindupMode=none  Kb=1  POutMin=[]  POutMax=[]  IOutMin=[]  IOutMax=[]  DOutMin=[]  DOutMax=[]  NOutMin=[]  NOutMax=[]  SumOutMin=[]  SumOutMax=[]  SaturationOutMin=[]  SaturationOutMax=[]  PParamMin=[]  PParamMax=[]  IParamMin=[]  IParamMax=[]  DParamMin=[]  DParamMax=[]  NParamMin=[]  NParamMax=[]  KbParamMin=[]  KbParamMax=[]  KtParamMin=[]  KtParamMax=[]  KbOutMin=[]  KbOutMax=[]  KtOutMin=[]  KtOutMax=[]  IntegratorOutMin=[]  IntegratorOutMax=[]  FilterOutMin=[]  FilterOutMax=[]  SumI1OutMin=[]  SumI1OutMax=[]  SumI2OutMin=[]  SumI2OutMax=[]  SumI3OutMin=[]  SumI3OutMax=[]  SumI4OutMin=[]  SumI4OutMax=[]  SumDOutMin=[]  SumDOutMax=[]  DifferentiatorOutMin=[]  DifferentiatorOutMax=[]  FilterDiffOutCoefMin=[]  FilterDiffOutCoefMax=[]  ReciprocalOutMin=[]  ReciprocalOutMax=[]  SumDenOutMin=[]  SumDenOutMax=[]  SumNumOutMin=[]  SumNumOutMax=[]  DivideOutMin=[]  DivideOutMax=[]  IntegratorContinuousStateAttributes=''  IntegratorStateMustResolveToSignalObject=off  IntegratorRTWStateStorageClass=Auto  FilterContinuousStateAttributes=''  FilterStateMustResolveToSignalObject=off  FilterRTWStateStorageClass=Auto  ParallelPVariant=InternalParameters  IdealPVariant=Disabled  IVariant=InternalParameters  DVariant=InternalParameters  IntegratorVariant=Continuous  SatVariant=Disabled  AWVariant=Passthrough  PCopyVariant=Disabled  TRVariant=Disabled  FdbkBlocksVariant=Forward  IdealPFdbkVariant=Disabled  SatFdbkVariant=Disabled  DerivativeFilterVariant=ContFilter  NVariant=InternalParameters  NCopyVariant=Disabled  FilterICVariant=InternalICsFilter  IntegratorICVariant=InternalICs  ExternalResetVariant=Disabled  TRSumVariant=Passthrough  SumFdbkVariant=Disabled  SumVariant=Sum_PID
  PID Controller2 : simulink/Continuous/PID Controller  Controller=PID  Form=Parallel  TimeDomain=Continuous-time  SampleTime=0.02  IntegratorMethod=Forward Euler  FilterMethod=Forward Euler  ControllerParametersSource=internal  P=0.2  I=0.02  D=0  UseFilter=on  N=100  TunerSelectOption=Transfer Function Based (PID Tuner App)  InitialConditionSource=internal  InitialConditionForIntegrator=0  InitialConditionForFilter=0  DifferentiatorICPrevScaledInput=0  ExternalReset=none  TrackingMode=off  Kt=1  LimitOutput=off  UpperSaturationLimit=inf  LowerSaturationLimit=-inf  LinearizeAsGain=on  AntiWindupMode=none  Kb=1  POutMin=[]  POutMax=[]  IOutMin=[]  IOutMax=[]  DOutMin=[]  DOutMax=[]  NOutMin=[]  NOutMax=[]  SumOutMin=[]  SumOutMax=[]  SaturationOutMin=[]  SaturationOutMax=[]  PParamMin=[]  PParamMax=[]  IParamMin=[]  IParamMax=[]  DParamMin=[]  DParamMax=[]  NParamMin=[]  NParamMax=[]  KbParamMin=[]  KbParamMax=[]  KtParamMin=[]  KtParamMax=[]  KbOutMin=[]  KbOutMax=[]  KtOutMin=[]  KtOutMax=[]  IntegratorOutMin=[]  IntegratorOutMax=[]  FilterOutMin=[]  FilterOutMax=[]  SumI1OutMin=[]  SumI1OutMax=[]  SumI2OutMin=[]  SumI2OutMax=[]  SumI3OutMin=[]  SumI3OutMax=[]  SumI4OutMin=[]  SumI4OutMax=[]  SumDOutMin=[]  SumDOutMax=[]  DifferentiatorOutMin=[]  DifferentiatorOutMax=[]  FilterDiffOutCoefMin=[]  FilterDiffOutCoefMax=[]  ReciprocalOutMin=[]  ReciprocalOutMax=[]  SumDenOutMin=[]  SumDenOutMax=[]  SumNumOutMin=[]  SumNumOutMax=[]  DivideOutMin=[]  DivideOutMax=[]  IntegratorContinuousStateAttributes=''  IntegratorStateMustResolveToSignalObject=off  IntegratorRTWStateStorageClass=Auto  FilterContinuousStateAttributes=''  FilterStateMustResolveToSignalObject=off  FilterRTWStateStorageClass=Auto  ParallelPVariant=InternalParameters  IdealPVariant=Disabled  IVariant=InternalParameters  DVariant=InternalParameters  IntegratorVariant=Continuous  SatVariant=Disabled  AWVariant=Passthrough  PCopyVariant=Disabled  TRVariant=Disabled  FdbkBlocksVariant=Forward  IdealPFdbkVariant=Disabled  SatFdbkVariant=Disabled  DerivativeFilterVariant=ContFilter  NVariant=InternalParameters  NCopyVariant=Disabled  FilterICVariant=InternalICsFilter  IntegratorICVariant=InternalICs  ExternalResetVariant=Disabled  TRSumVariant=Passthrough  SumFdbkVariant=Disabled  SumVariant=Sum_PID
  RT_xy : Gain  Gain=0.95
  RT_z : Gain
  Scope : Scope
  Scope1 : Scope
  Sum : Sum  Inputs=|++
  Sum1 : Sum  Inputs=|+-
  Sum2 : Sum  Inputs=|+-
  Sum3 : Sum  Inputs=|+-
  Terminator : Terminator
  Vertical thrust compensation : Subsystem
  xiDot1 : InportShadow  Port=3  PortDimensions=3
  qd : Outport
  thrust_sp : Outport  Port=2
  yawRateDes : Outport  Port=3
  horThrust : Outport  Port=4  PortDimensions=2
  wires:
  Vertical thrust compensation/2(" horThrustBody") -> horThrust/1
  Horizontal thrust control/1(" horThrust") -> Vertical thrust compensation/2("horThrust "), Scope/1
  Constant4/1 -> Horizontal thrust control/3(controller)
  xiDot1/1 -> Horizontal thrust control/2("xiDot ")
  Constant3/1 -> Vertical thrust compensation/3(compType)
  Vertical thrust compensation/1(" vertThurstComp") -> Mux/2, Sum/2
  q/1 -> Vertical thrust compensation/1("q ")
  Mux/1 -> Scope1/1
  Sum/1 -> Gain/1
  PID Controller2/1 -> Sum2/1
  PID Controller1/1 -> Mux1/2
  PID Controller/1 -> Mux1/1
  Demux/3 -> PID Controller2/1
  Demux/2 -> PID Controller1/1
  Demux/1 -> PID Controller/1
  Sum1/1 -> Demux3/1, Horizontal thrust control/1("xiErr ")
  Gain/1 -> thrust_sp/1
  Sum2/1 -> Mux1/3
  Constant2/1 -> Sum2/2
  RT_z/1 -> Mux6/3
  Constant/1 -> MATLAB Function/2(yaw_sp)
  MATLAB Function/2(thrust_sp) -> Sum/1, Mux/1
  Mux1/1 -> MATLAB Function/1(thr_sp)
  Sum3/1 -> Demux/1
  xiDot/1 -> Sum3/2
  nuBody/1 -> Terminator/1
  xiDes/1 -> Sum1/1
  xi/1 -> Sum1/2
  Demux3/1 -> Mux3/1
  Demux3/2 -> Mux3/2
  Mux3/1 -> RT_xy/1
  Demux3/3 -> RT_z/1
  RT_xy/1 -> Demux6/1
  Mux6/1 -> Sum3/1
  Demux6/2 -> Mux6/2
  Constant1/1 -> yawRateDes/1
  Demux6/1 -> Mux6/1
  MATLAB Function/1(q_sp) -> qd/1

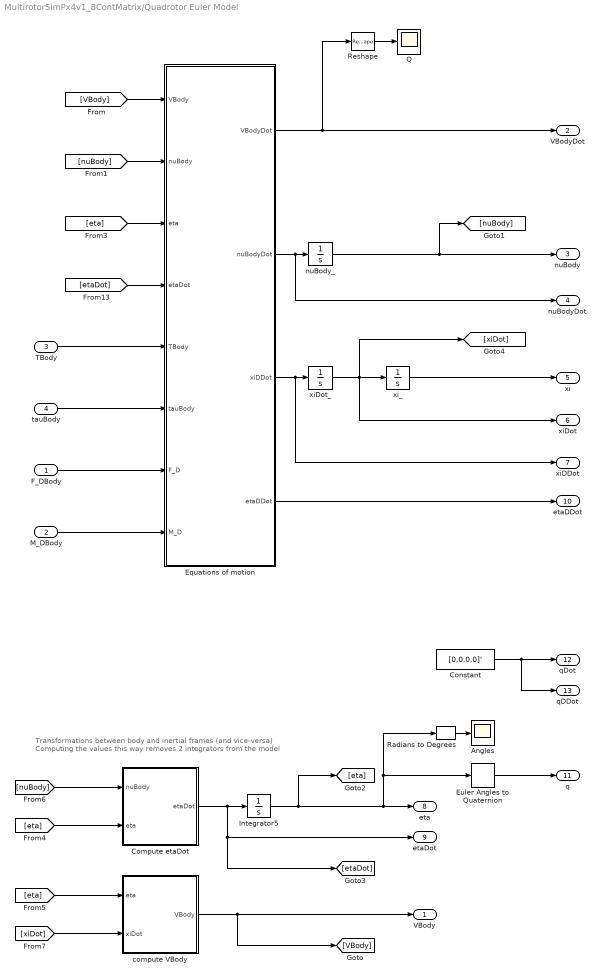
== system MultirotorSimPx4v1_8ContMatrix/Quadrotor Euler Model ==
  note: Transformations between body and inertial frames (and vice-versa)
      | Computing the values this way removes 2 integrators from the model
  F_DBody : Inport  Unit=N
  M_DBody : Inport  Port=2  Unit=N*m
  TBody : Inport  Port=3  Unit=N
  tauBody : Inport  Port=4  Unit=N*m
  Angles : Scope
  Compute etaDot : MATLAB Function  TreatAsAtomicUnit=on
  Constant : Constant  Value=[0,0,0,0]'
  Equations of motion : MATLAB Function  TreatAsAtomicUnit=on
  Euler Angles to Quaternion : QuaternionLibrary/Euler Angles to Quaternion
  Integrator5 : Integrator  InitialCondition=Initial.ETA  ContinuousStateAttributes='eta'
  Q : Scope
  Radians to Degrees : simulink_extras/Transformations/Radians to Degrees
  Reshape : Reshape  OutputDimensionality=Column vector (2-D)
  compute VBody : MATLAB Function  TreatAsAtomicUnit=on
  nuBody_ : Integrator  InitialCondition=Initial.NU_BODY  ContinuousStateAttributes='nuBody'
  xiDot_ : Integrator  InitialCondition=Initial.XI_DOT  ContinuousStateAttributes='xiDot'
  xi_ : Integrator  InitialCondition=Initial.XI  ContinuousStateAttributes='xi'
  VBody : Outport  Unit=m/s
  VBodyDot : Outport  Port=2  Unit=m/s^2
  nuBody : Outport  Port=3  Unit=rad/s
  nuBodyDot : Outport  Port=4  Unit=rad/s^2
  xi : Outport  Port=5  Unit=m
  xiDot : Outport  Port=6  Unit=m/s
  xiDDot : Outport  Port=7  Unit=m/s^2
  eta : Outport  Port=8  Unit=rad
  etaDot : Outport  Port=9  Unit=rad/s
  etaDDot : Outport  Port=10  Unit=rad/s^2
  q : Outport  Port=11
  qDot : Outport  Port=12
  qDDot : Outport  Port=13
  wires:
  Radians to Degrees/1 -> Angles/1
  Constant/1 -> qDot/1, qDDot/1
  Euler Angles to Quaternion/1 -> q/1
  Integrator5/1 -> [eta], eta/1, Euler Angles to Quaternion/1, Radians to Degrees/1
  Compute etaDot/1(etaDot) -> Integrator5/1, [etaDot], etaDot/1
  [eta] -> Compute etaDot/2(eta)
  compute VBody/1(VBody) -> [VBody], VBody/1
  [eta] -> compute VBody/1(eta)
  [nuBody] -> Compute etaDot/1(nuBody)
  [xiDot] -> compute VBody/2(xiDot)
  [etaDot] -> Equations of motion/4(etaDot)
  xiDot_/1 -> xiDot/1, [xiDot], xi_/1
  Reshape/1 -> Q/1
  Equations of motion/4(etaDDot) -> etaDDot/1
  [eta] -> Equations of motion/3(eta)
  Equations of motion/2(nuBodyDot) -> nuBodyDot/1, nuBody_/1
  nuBody_/1 -> nuBody/1, [nuBody]
  M_DBody/1 -> Equations of motion/8(M_D)
  F_DBody/1 -> Equations of motion/7(F_D)
  Equations of motion/3(xiDDot) -> xiDDot/1, xiDot_/1
  TBody/1 -> Equations of motion/5(TBody)
  tauBody/1 -> Equations of motion/6(tauBody)
  [VBody] -> Equations of motion/1(VBody)
  [nuBody] -> Equations of motion/2(nuBody)
  xi_/1 -> xi/1
  Equations of motion/1(VBodyDot) -> VBodyDot/1, Reshape/1

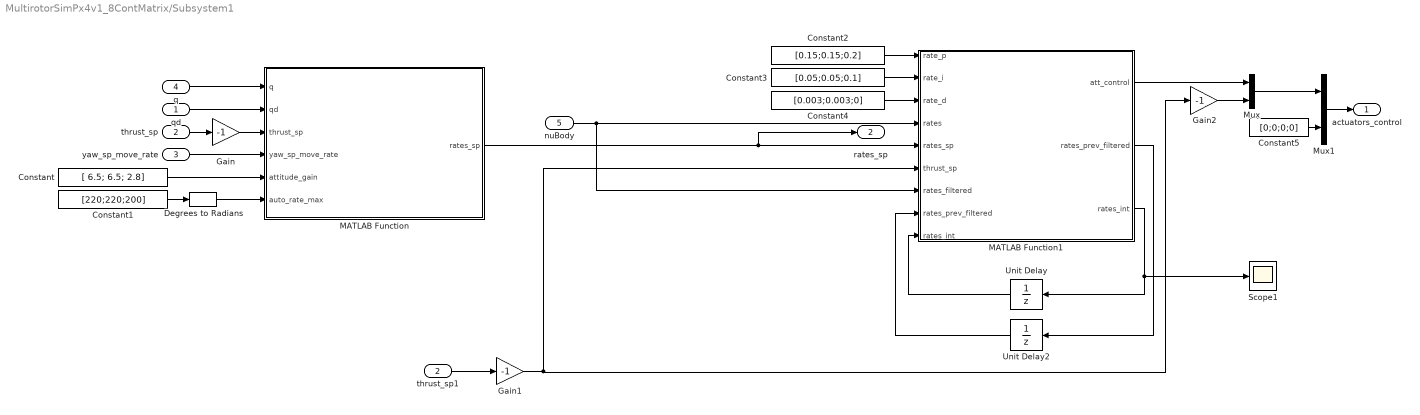
== system MultirotorSimPx4v1_8ContMatrix/Subsystem1 ==
  qd : Inport
  thrust_sp : Inport  Port=2
  yaw_sp_move_rate : Inport  Port=3
  q : Inport  Port=4
  nuBody : Inport  Port=5
  Constant : Constant  Value=[ 6.5; 6.5; 2.8]
  Constant1 : Constant  Value=[220;220;200]
  Constant2 : Constant  Value=[0.15;0.15;0.2]
  Constant3 : Constant  Value=[0.05;0.05;0.1]
  Constant4 : Constant  Value=[0.003;0.003;0]
  Constant5 : Constant  Value=[0;0;0;0]
  Degrees to Radians : simulink_extras/Transformations/Degrees to Radians
  Gain : Gain  Gain=-1
  Gain1 : Gain  Gain=-1
  Gain2 : Gain  Gain=-1
  MATLAB Function : MATLAB Function  TreatAsAtomicUnit=on  SystemSampleTime=1/250
  MATLAB Function1 : MATLAB Function  TreatAsAtomicUnit=on  SystemSampleTime=1/250
  Mux : Mux  Inputs=2
  Mux1 : Mux  Inputs=2
  Scope1 : Scope
  Unit Delay : UnitDelay  SampleTime=1/250  StateName=rates_int
  Unit Delay2 : UnitDelay  SampleTime=1/250  StateName=rates_prev_filtered
  thrust_sp1 : InportShadow  Port=2
  actuators_control : Outport
  rates_sp : Outport  Port=2
  wires:
  qd/1 -> MATLAB Function/2(qd)
  q/1 -> MATLAB Function/1(q)
  Constant/1 -> MATLAB Function/5(attitude_gain)
  Constant1/1 -> Degrees to Radians/1
  Degrees to Radians/1 -> MATLAB Function/6(auto_rate_max)
  yaw_sp_move_rate/1 -> MATLAB Function/4(yaw_sp_move_rate)
  Constant4/1 -> MATLAB Function1/3(rate_d)
  Constant3/1 -> MATLAB Function1/2(rate_i)
  Constant2/1 -> MATLAB Function1/1(rate_p)
  MATLAB Function1/1(att_control) -> Mux/1
  nuBody/1 -> MATLAB Function1/7(rates_filtered), MATLAB Function1/4(rates)
  Unit Delay/1 -> MATLAB Function1/9("rates_int ")
  MATLAB Function1/3(rates_int) -> Unit Delay/1, Scope1/1
  Mux/1 -> Mux1/1
  Unit Delay2/1 -> MATLAB Function1/8("rates_prev_filtered ")
  MATLAB Function1/2(rates_prev_filtered) -> Unit Delay2/1
  thrust_sp1/1 -> Gain1/1
  Constant5/1 -> Mux1/2
  Mux1/1 -> actuators_control/1
  thrust_sp/1 -> Gain/1
  MATLAB Function/1(rates_sp) -> MATLAB Function1/5(rates_sp), rates_sp/1
  Gain/1 -> MATLAB Function/3(thrust_sp)
  Gain1/1 -> Gain2/1, MATLAB Function1/6(thrust_sp)
  Gain2/1 -> Mux/2

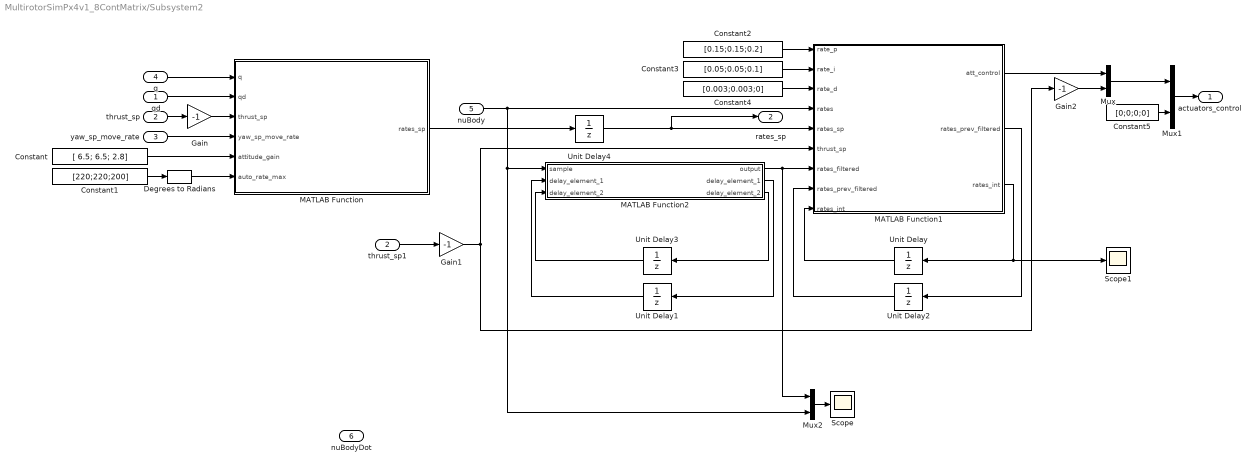
== system MultirotorSimPx4v1_8ContMatrix/Subsystem2 ==
  qd : Inport
  thrust_sp : Inport  Port=2
  yaw_sp_move_rate : Inport  Port=3
  q : Inport  Port=4
  nuBody : Inport  Port=5
  nuBodyDot : Inport  Port=6
  Constant : Constant  Value=[ 6.5; 6.5; 2.8]
  Constant1 : Constant  Value=[220;220;200]
  Constant2 : Constant  Value=[0.15;0.15;0.2]
  Constant3 : Constant  Value=[0.05;0.05;0.1]
  Constant4 : Constant  Value=[0.003;0.003;0]
  Constant5 : Constant  Value=[0;0;0;0]
  Degrees to Radians : simulink_extras/Transformations/Degrees to Radians
  Gain : Gain  Gain=-1
  Gain1 : Gain  Gain=-1
  Gain2 : Gain  Gain=-1
  MATLAB Function : MATLAB Function  TreatAsAtomicUnit=on  SystemSampleTime=1/250
  MATLAB Function1 : MATLAB Function  TreatAsAtomicUnit=on  SystemSampleTime=1/250
  MATLAB Function2 : MATLAB Function  TreatAsAtomicUnit=on  SystemSampleTime=1/250
  Mux : Mux  Inputs=2
  Mux1 : Mux  Inputs=2
  Mux2 : Mux  Inputs=2
  Scope : Scope
  Scope1 : Scope
  Unit Delay : UnitDelay  SampleTime=1/250  StateName=rates_int
  Unit Delay1 : UnitDelay  SampleTime=1/250  StateName=lp_filters_d_delay_element_1
  Unit Delay2 : UnitDelay  SampleTime=1/250  StateName=rates_prev_filtered
  Unit Delay3 : UnitDelay  SampleTime=1/250  StateName=lp_filters_d_delay_element_2
  Unit Delay4 : UnitDelay  SampleTime=1/250  StateName=rates_sp
  thrust_sp1 : InportShadow  Port=2
  actuators_control : Outport
  rates_sp : Outport  Port=2
  wires:
  qd/1 -> MATLAB Function/2(qd)
  q/1 -> MATLAB Function/1(q)
  Constant/1 -> MATLAB Function/5(attitude_gain)
  Constant1/1 -> Degrees to Radians/1
  Degrees to Radians/1 -> MATLAB Function/6(auto_rate_max)
  yaw_sp_move_rate/1 -> MATLAB Function/4(yaw_sp_move_rate)
  Constant4/1 -> MATLAB Function1/3(rate_d)
  Constant3/1 -> MATLAB Function1/2(rate_i)
  Constant2/1 -> MATLAB Function1/1(rate_p)
  MATLAB Function/1(rates_sp) -> Unit Delay4/1
  MATLAB Function1/1(att_control) -> Mux/1
  nuBody/1 -> MATLAB Function1/4(rates), MATLAB Function2/1(sample), Mux2/2
  Unit Delay/1 -> MATLAB Function1/9("rates_int ")
  MATLAB Function1/3(rates_int) -> Unit Delay/1, Scope1/1
  Unit Delay1/1 -> MATLAB Function2/2("delay_element_1 ")
  Mux/1 -> Mux1/1
  Unit Delay2/1 -> MATLAB Function1/8("rates_prev_filtered ")
  MATLAB Function1/2(rates_prev_filtered) -> Unit Delay2/1
  Unit Delay3/1 -> MATLAB Function2/3("delay_element_2 ")
  MATLAB Function2/3(delay_element_2) -> Unit Delay3/1
  MATLAB Function2/2(delay_element_1) -> Unit Delay1/1
  thrust_sp1/1 -> Gain1/1
  Constant5/1 -> Mux1/2
  Mux1/1 -> actuators_control/1
  thrust_sp/1 -> Gain/1
  Mux2/1 -> Scope/1
  Unit Delay4/1 -> MATLAB Function1/5(rates_sp), rates_sp/1
  Gain/1 -> MATLAB Function/3(thrust_sp)
  Gain1/1 -> Gain2/1, MATLAB Function1/6(thrust_sp)
  Gain2/1 -> Mux/2
  MATLAB Function2/1(output) -> Mux2/1, MATLAB Function1/7(rates_filtered)

== system MultirotorSimPx4v1_8ContMatrix/Attitude Controller/Pitch rate PID ==
  ref : Inport
  meas : Inport  Port=2
  Add : Sum  Inputs=++-
  D : Gain  Gain=PID_D
  D filter : TransferFcn  Numerator=[(PID_FC*2*pi)^2 0]  Denominator="[1 2*(PID_FC*2*pi)*0.68  (PID_FC*2*pi)^2]"  ContinuousStateAttributes=PID_D_STATENAME
  I : Gain  Gain=PID_I
  Integrator1 : Integrator  LimitOutput=on  UpperSaturationLimit=0.3  LowerSaturationLimit=-0.3  ContinuousStateAttributes=PID_I_STATENAME
  P : Gain  Gain=PID_P
  Sum : Sum  Inputs=|+-
  Out : Outport
  wires:
  meas/1 -> Sum/2, D filter/1
  ref/1 -> Sum/1
  I/1 -> Integrator1/1
  D/1 -> Add/3
  Sum/1 -> I/1, P/1
  D filter/1 -> D/1
  Integrator1/1 -> Add/2
  P/1 -> Add/1
  Add/1 -> Out/1

== system MultirotorSimPx4v1_8ContMatrix/Attitude Controller/Roll rate PID ==
  ref : Inport
  meas : Inport  Port=2
  Add : Sum  Inputs=++-
  D : Gain  Gain=PID_D
  D filter : TransferFcn  Numerator=[(PID_FC*2*pi)^2 0]  Denominator="[1 2*(PID_FC*2*pi)*0.68  (PID_FC*2*pi)^2]"  ContinuousStateAttributes=PID_D_STATENAME
  I : Gain  Gain=PID_I
  Integrator1 : Integrator  LimitOutput=on  UpperSaturationLimit=0.3  LowerSaturationLimit=-0.3  ContinuousStateAttributes=PID_I_STATENAME
  P : Gain  Gain=PID_P
  Sum : Sum  Inputs=|+-
  Out : Outport
  wires:
  Add/1 -> Out/1
  P/1 -> Add/1
  Integrator1/1 -> Add/2
  D filter/1 -> D/1
  Sum/1 -> P/1, I/1
  D/1 -> Add/3
  I/1 -> Integrator1/1
  ref/1 -> Sum/1
  meas/1 -> D filter/1, Sum/2

== system MultirotorSimPx4v1_8ContMatrix/Attitude Controller/Yaw rate PID ==
  ref : Inport
  meas : Inport  Port=2
  Add : Sum  Inputs=++-
  D : Gain  Gain=PID_D
  D filter : TransferFcn  Numerator=[(PID_FC*2*pi)^2 0]  Denominator="[1 2*(PID_FC*2*pi)*0.68  (PID_FC*2*pi)^2]"  ContinuousStateAttributes=PID_D_STATENAME
  I : Gain  Gain=PID_I
  Integrator1 : Integrator  LimitOutput=on  UpperSaturationLimit=0.3  LowerSaturationLimit=-0.3  ContinuousStateAttributes=PID_I_STATENAME
  P : Gain  Gain=PID_P
  Sum : Sum  Inputs=|+-
  Out : Outport
  wires:
  Add/1 -> Out/1
  P/1 -> Add/1
  Integrator1/1 -> Add/2
  D filter/1 -> D/1
  Sum/1 -> P/1, I/1
  D/1 -> Add/3
  I/1 -> Integrator1/1
  ref/1 -> Sum/1
  meas/1 -> D filter/1, Sum/2
